simulink model "if_else_statement"  (R2021a)
settings: Solver=VariableStepAuto  StartTime=0.0  StopTime=10.0  RelTol=1e-3
settings Model: Creator=Acer  LastModifiedBy=Acer

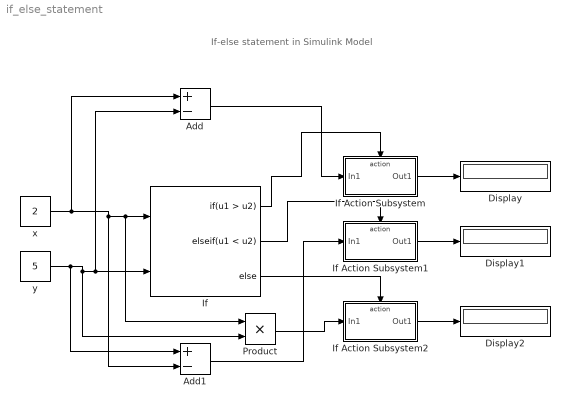
== system if_else_statement ==
  note: If-else statement in Simulink Model
  Add : Sum  Inputs=+-
  Add1 : Sum  Inputs=+-
  Display : Display
  Display1 : Display
  Display2 : Display
  If : If  NumInputs=2  IfExpression=u1 > u2  ElseIfExpressions=u1 < u2
  If Action Subsystem : Subsystem  TreatAsAtomicUnit=on
  If Action Subsystem1 : Subsystem  TreatAsAtomicUnit=on
  If Action Subsystem2 : Subsystem  TreatAsAtomicUnit=on
  Product : Product
  x : Constant  Value=2
  y : Constant  Value=5
  wires:
  x/1 -> Add/1, Add1/2, Product/1, If/1
  y/1 -> Add1/1, Product/2, Add/2, If/2
  Add/1 -> If Action Subsystem/1(In1)
  If/1 -> If Action Subsystem/Action
  If Action Subsystem/1(Out1) -> Display/1
  If Action Subsystem1/1(Out1) -> Display1/1
  Add1/1 -> If Action Subsystem1/1(In1)
  If/2 -> If Action Subsystem1/Action
  If Action Subsystem2/1(Out1) -> Display2/1
  Product/1 -> If Action Subsystem2/1(In1)
  If/3 -> If Action Subsystem2/Action

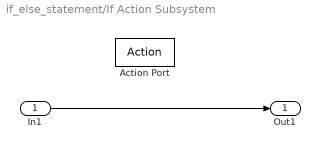
== system if_else_statement/If Action Subsystem ==
  In1 : Inport
  Action Port : ActionPort  ActionPortLabel=if(u1 > u2)
  Out1 : Outport
  wires:
  In1/1 -> Out1/1

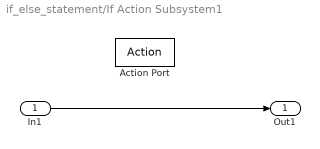
== system if_else_statement/If Action Subsystem1 ==
  In1 : Inport
  Action Port : ActionPort  ActionPortLabel=elseif(u1 < u2)
  Out1 : Outport
  wires:
  In1/1 -> Out1/1

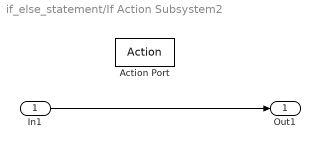
== system if_else_statement/If Action Subsystem2 ==
  In1 : Inport
  Action Port : ActionPort  ActionPortLabel=else
  Out1 : Outport
  wires:
  In1/1 -> Out1/1
